simulink model "UAV_control"  (R2023a)
settings: Solver=FixedStepAuto  StartTime=0.0  StopTime=20  FixedStep=0.01  RelTol=1e-3
InitFcn:
  | parameters_UAV
values from neighbouring files (symbols this model uses):
  attitudeInit = [0;0;0]    [parameters_UAV.m]
  b = m*g/(4*w0r^2)    (= 1.31218568726e-05)    [parameters_UAV.m]
  d = 1.218100e-07    (= 1.2181e-07)    [parameters_UAV.m]
  g = 9.81    [parameters_UAV.m]
  I = diag([Ix, Iy, Iz])    [parameters_UAV.m]
  Jm = 12*10^-6    (= 1.2e-05)    [parameters_UAV.m]
  Ke = Kt    (= 0.00502594557132)    [parameters_UAV.m]
  Kp1P = Iy*etaP*wnP/(Kth*L)    (= 0.0922548996874)    [parameters_UAV.m]
  Kp1R = Ix*etaR*wnR/(Kth*L)    (= 0.0956695521884)    [parameters_UAV.m]
  Kp1x = 2*m*etax*wnx/U1    (= 0.203873598369)    [parameters_UAV.m]
  Kp1Y = Iz*etaY*wnY/(2*Kd)    (= 0.791166525164)    [parameters_UAV.m]
  Kp1y = 2*m*etay*wny/U1    (= 0.203873598369)    [parameters_UAV.m]
  Kp1z = m*etaz*wnz/(2*Kth)    (= 2.43380373272)    [parameters_UAV.m]
  Kp2P = Iy*wnP^2/(2*Kth*L*Kp1P)    (= 4.28571428571)    [parameters_UAV.m]
  Kp2R = Ix*wnR^2/(2*Kth*L*Kp1R)    (= 4.28571428571)    [parameters_UAV.m]
  Kp2x = m*wnx^2/(U1*Kp1x)    (= 0.5)    [parameters_UAV.m]
  Kp2Y = Iz*wnY^2/(4*Kd*Kp1Y)    (= 2.85714285714)    [parameters_UAV.m]
  Kp2y = m*wny^2/(U1*Kp1y)    (= 0.5)    [parameters_UAV.m]
  Kp2z = m*wnz^2/(4*Kth*Kp1z)    (= 0.333333333333)    [parameters_UAV.m]
  Kt = 1/(1900/60*2*pi)    (= 0.00502594557132)    [parameters_UAV.m]
  L = 0.211    [parameters_UAV.m]
  m = 1.362    [parameters_UAV.m]
  MotorSpeedInit = 0    [parameters_UAV.m]
  omegaInit = [0;0;0]    [parameters_UAV.m]
  posInit = [0;0;0]    [parameters_UAV.m]
  Ra = 0.128    [parameters_UAV.m]
  u0 = (w0-1075)/7525    (= 0.497408637874)    [parameters_UAV.m]
  velInit = [0;0;0]    [parameters_UAV.m]
settings Model: Creator=THETRUNG  LastModifiedBy=ducdu
settings SolverCC: AlgebraicLoopSolver=TrustRegion
settings OptimizationCC: UseRowMajorAlgorithm=on
settings DebuggingCC: UnconnectedInputMsg=warning  UnconnectedOutputMsg=warning  UnconnectedLineMsg=warning
settings ModelReferenceCC: EnableRefExpFcnMdlSchedulingChecks=on
settings SFSimCC: CustomCodeUndefinedFunction=UseInterfaceOnly

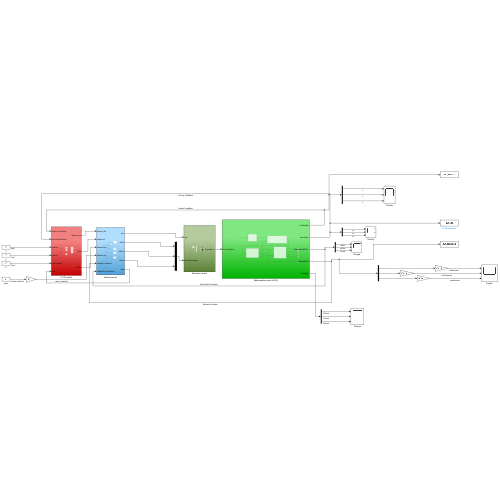
[thumbnail: Simulink's stored preview of the top-level diagram]
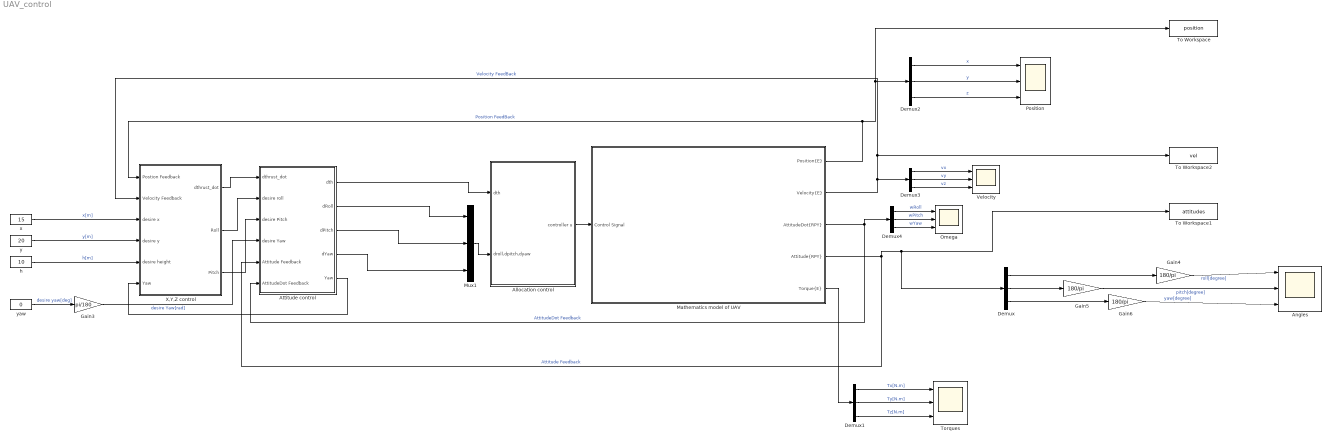
== system UAV_control ==
  "Allocation control " : Subsystem
  Angles : Scope  NumInputPorts=3
  Attitude control : Subsystem
  Demux{,1..4} (5 alike) : Demux  Outputs=3
  Gain3 : Gain  Gain=pi/180
  Gain4 : Gain  Gain=180/pi
  Gain5 : Gain  Gain=180/pi
  Gain6 : Gain  Gain=180/pi
  Mathematics model of UAV : Subsystem
  Mux1 : Mux  Inputs=3
  Omega : Scope  NumInputPorts=3
  Position : Scope  NumInputPorts=3
  To Workspace : ToWorkspace  VariableName=position  SampleTime=1
  To Workspace1 : ToWorkspace  VariableName=attitudes  SampleTime=1
  To Workspace2 : ToWorkspace  VariableName=vel  SampleTime=1
  Torques : Scope  NumInputPorts=3
  Velocity : Scope  NumInputPorts=3
  X,Y,Z control : Subsystem
  h : Constant  Value=10
  x : Constant  Value=15
  y : Constant  Value=20
  "yaw " : Constant  Value=0
  wires:
  Demux/1 -> Gain4/1
  Demux/2 -> Gain5/1
  Demux/3 -> Gain6/1
  Demux1/1 -> Torques/1  "Tx[N.m]"
  Demux1/2 -> Torques/2  "Ty[N.m]"
  Demux1/3 -> Torques/3  "Tz[N.m]"
  Demux2/3 -> Position/3  "z"
  Demux2/1 -> Position/1  "x"
  Demux2/2 -> Position/2  "y"
  "yaw "/1 -> Gain3/1  "desire yaw[deg]"
  Demux3/3 -> Velocity/3  "vz"
  Demux3/1 -> Velocity/1  "vx"
  Demux3/2 -> Velocity/2  "vy"
  Demux4/2 -> Omega/2  "wPitch"
  Demux4/1 -> Omega/1  "wRoll"
  Demux4/3 -> Omega/3  "wYaw"
  "Allocation control "/1("controller u ") -> Mathematics model of UAV/1(Control Signal)
  Mathematics model of UAV/1("Position{E} ") -> X,Y,Z control/1(Postion Feedback), Demux2/1, To Workspace/1  "Position FeedBack"
  Mathematics model of UAV/5("Torque{E} ") -> Demux1/1
  Mathematics model of UAV/2("Velocity{E} ") -> To Workspace2/1, X,Y,Z control/2(Velocity Feedback), Demux3/1  "Velocity FeedBack"
  Mathematics model of UAV/3("AttitudeDot{RPY} ") -> Demux4/1, Attitude control/6(AttitudeDot Feedback)  "AttitudeDot Feedback"
  Mux1/1 -> "Allocation control "/2("droll,dpitch,dyaw ")
  Mathematics model of UAV/4("Attitude{RPY}") -> To Workspace1/1, Demux/1, Attitude control/5(Attitude Feedback)  "Attitude Feedback"
  Attitude control/2(dRoll) -> Mux1/1
  Attitude control/3(dPitch) -> Mux1/2
  Attitude control/4(dYaw) -> Mux1/3
  X,Y,Z control/1(dthrust_dot) -> Attitude control/1(dthrust_dot)
  Gain4/1 -> Angles/1  "roll[degree]"
  Gain5/1 -> Angles/2  "pitch[degree]"
  Gain6/1 -> Angles/3  "yaw[degree]"
  x/1 -> X,Y,Z control/3(desire x)  "x[m]"
  y/1 -> X,Y,Z control/4(desire y)  "y[m]"
  h/1 -> X,Y,Z control/5(desire height)  "h[m]"
  Attitude control/1("dth ") -> "Allocation control "/1(dth)
  X,Y,Z control/2(Roll) -> Attitude control/2(desire roll)
  X,Y,Z control/3(Pitch) -> Attitude control/3(desire Pitch)
  Gain3/1 -> Attitude control/4(desire Yaw)  "desire Yaw[rad]"
  Attitude control/5(Yaw) -> X,Y,Z control/6(Yaw)

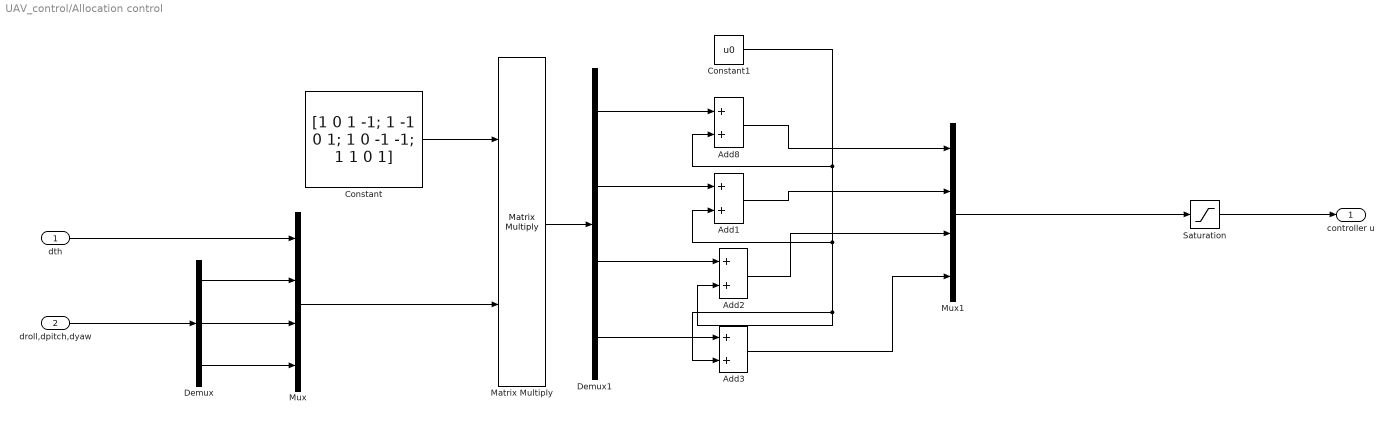
== system UAV_control/Allocation control  ==
  dth : Inport
  "droll,dpitch,dyaw " : Inport  Port=2
  Add{1..3,8} (4 alike) : Sum
  Constant : Constant  Value=[1 0 1 -1; 1 -1 0 1; 1 0 -1 -1; 1 1 0 1]
  Constant1 : Constant  Value=u0
  Demux : Demux  Outputs=3
  Demux1 : Demux
  Matrix Multiply : Product  Multiplication=Matrix(*)
  Mux : Mux
  Mux1 : Mux
  Saturation : Saturate  UpperLimit=1  LowerLimit=0
  "controller u " : Outport  VectorParamsAs1DForOutWhenUnconnected=off
  wires:
  "droll,dpitch,dyaw "/1 -> Demux/1
  Demux/3 -> Mux/4
  Demux/2 -> Mux/3
  Demux/1 -> Mux/2
  dth/1 -> Mux/1
  Constant/1 -> Matrix Multiply/1
  Mux/1 -> Matrix Multiply/2
  Matrix Multiply/1 -> Demux1/1
  Demux1/1 -> Add8/1
  Demux1/2 -> Add1/1
  Demux1/3 -> Add2/1
  Demux1/4 -> Add3/1
  Constant1/1 -> Add8/2, Add1/2, Add2/2, Add3/2
  Add8/1 -> Mux1/1
  Add1/1 -> Mux1/2
  Add2/1 -> Mux1/3
  Add3/1 -> Mux1/4
  Mux1/1 -> Saturation/1
  Saturation/1 -> "controller u "/1

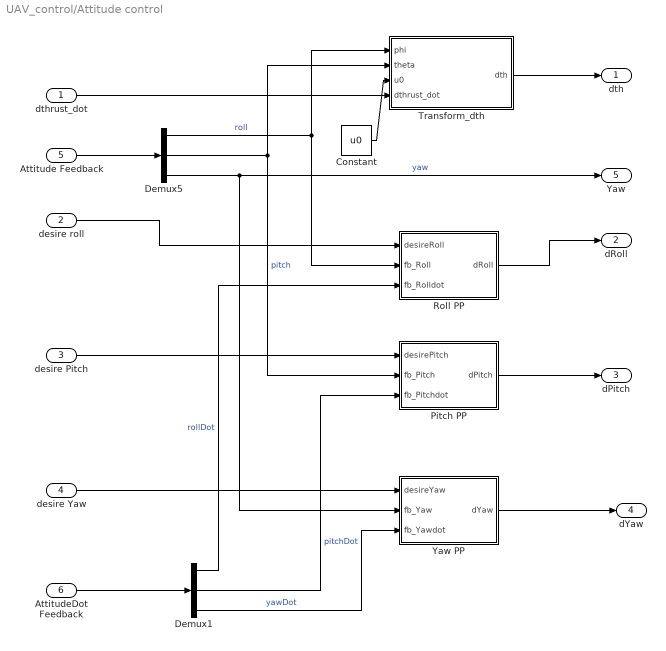
== system UAV_control/Attitude control ==
  dthrust_dot : Inport
  desire roll : Inport  Port=2
  desire Pitch : Inport  Port=3
  desire Yaw : Inport  Port=4
  Attitude Feedback : Inport  Port=5
  AttitudeDot Feedback : Inport  Port=6
  Constant : Constant  Value=u0
  Demux1 : Demux  Outputs=3
  Demux5 : Demux  Outputs=3
  Pitch PP : Subsystem
  "Roll PP " : Subsystem
  Transform_dth : MATLAB Function  TreatAsAtomicUnit=on
  Yaw PP : Subsystem
  "dth " : Outport  VectorParamsAs1DForOutWhenUnconnected=off
  dRoll : Outport  Port=2  VectorParamsAs1DForOutWhenUnconnected=off
  dPitch : Outport  Port=3  VectorParamsAs1DForOutWhenUnconnected=off
  dYaw : Outport  Port=4  VectorParamsAs1DForOutWhenUnconnected=off
  Yaw : Outport  Port=5  VectorParamsAs1DForOutWhenUnconnected=off
  wires:
  Demux5/3 -> Yaw/1, Yaw PP/2(fb_Yaw)  "yaw"
  Demux5/1 -> Transform_dth/1(phi), "Roll PP "/2(fb_Roll)  "roll"
  desire roll/1 -> "Roll PP "/1("desireRoll ")
  Demux5/2 -> Transform_dth/2(theta), Pitch PP/2(fb_Pitch)  "pitch"
  Attitude Feedback/1 -> Demux5/1
  "Roll PP "/1("dRoll ") -> dRoll/1
  Pitch PP/1("dPitch ") -> dPitch/1
  Yaw PP/1("dYaw ") -> dYaw/1
  desire Pitch/1 -> Pitch PP/1("desirePitch ")
  desire Yaw/1 -> Yaw PP/1("desireYaw ")
  Demux1/1 -> "Roll PP "/3(fb_Rolldot)  "rollDot"
  AttitudeDot Feedback/1 -> Demux1/1
  Demux1/3 -> Yaw PP/3(fb_Yawdot)  "yawDot"
  Demux1/2 -> Pitch PP/3(fb_Pitchdot)  "pitchDot"
  Transform_dth/1(dth) -> "dth "/1
  dthrust_dot/1 -> Transform_dth/4(dthrust_dot)
  Constant/1 -> Transform_dth/3(u0)

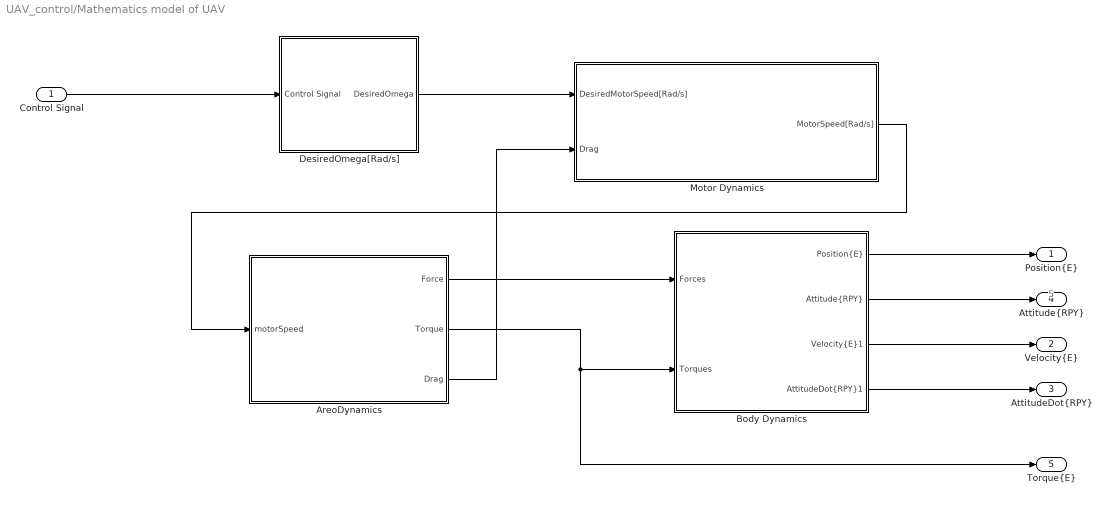
== system UAV_control/Mathematics model of UAV ==
  note: 5
  Control Signal : Inport
  "AreoDynamics " : Subsystem
  "Body Dynamics " : Subsystem
  DesiredOmega[Rad/s] : Subsystem
  Motor Dynamics : Subsystem
  "Position{E} " : Outport  VectorParamsAs1DForOutWhenUnconnected=off
  "Velocity{E} " : Outport  Port=2  VectorParamsAs1DForOutWhenUnconnected=off
  "AttitudeDot{RPY} " : Outport  Port=3  VectorParamsAs1DForOutWhenUnconnected=off
  "Attitude{RPY}" : Outport  Port=4  VectorParamsAs1DForOutWhenUnconnected=off
  "Torque{E} " : Outport  Port=5  VectorParamsAs1DForOutWhenUnconnected=off
  wires:
  "AreoDynamics "/1(Force) -> "Body Dynamics "/1("Forces ")
  Control Signal/1 -> DesiredOmega[Rad/s]/1(Control Signal)
  Motor Dynamics/1(MotorSpeed[Rad/s]) -> "AreoDynamics "/1(motorSpeed)
  "AreoDynamics "/2(Torque) -> "Torque{E} "/1, "Body Dynamics "/2("Torques ")
  "Body Dynamics "/4("AttitudeDot{RPY}1") -> "AttitudeDot{RPY} "/1
  DesiredOmega[Rad/s]/1(DesiredOmega) -> Motor Dynamics/1(DesiredMotorSpeed[Rad/s])
  "Body Dynamics "/2("Attitude{RPY}") -> "Attitude{RPY}"/1
  "AreoDynamics "/3("Drag ") -> Motor Dynamics/2("Drag ")
  "Body Dynamics "/1("Position{E}") -> "Position{E} "/1
  "Body Dynamics "/3("Velocity{E}1") -> "Velocity{E} "/1

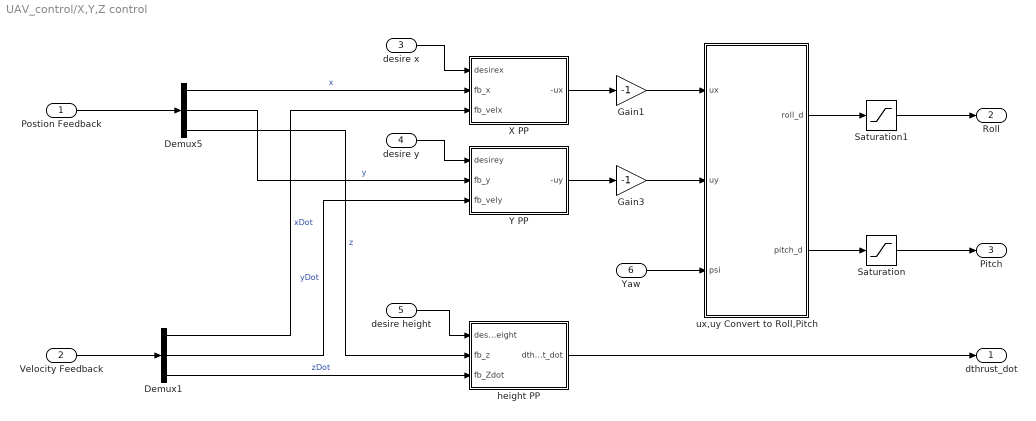
== system UAV_control/X,Y,Z control ==
  Postion Feedback : Inport
  Velocity Feedback : Inport  Port=2
  desire x : Inport  Port=3
  desire y : Inport  Port=4
  desire height : Inport  Port=5
  Yaw : Inport  Port=6
  Demux1 : Demux  Outputs=3
  Demux5 : Demux  Outputs=3
  Gain1 : Gain  Gain=-1  ParamDataTypeStr=double
  Gain3 : Gain  Gain=-1  ParamDataTypeStr=double
  Saturation : Saturate  UpperLimit=pi/8  LowerLimit=-pi/8
  Saturation1 : Saturate  UpperLimit=pi/8  LowerLimit=-pi/8
  "X PP " : Subsystem
  "Y PP " : Subsystem
  "height PP " : Subsystem
  ux,uy Convert to Roll,Pitch : MATLAB Function  TreatAsAtomicUnit=on
  dthrust_dot : Outport  VectorParamsAs1DForOutWhenUnconnected=off
  Roll : Outport  Port=2  OutDataTypeStr=double  VectorParamsAs1DForOutWhenUnconnected=off
  Pitch : Outport  Port=3  OutDataTypeStr=double  VectorParamsAs1DForOutWhenUnconnected=off
  wires:
  Demux5/3 -> "height PP "/2(fb_z)  "z"
  Demux5/1 -> "X PP "/2(fb_x)  "x"
  desire x/1 -> "X PP "/1("desirex ")
  Demux5/2 -> "Y PP "/2(fb_y)  "y"
  Postion Feedback/1 -> Demux5/1
  "Y PP "/1("-uy ") -> Gain3/1
  "height PP "/1("dthrust_dot ") -> dthrust_dot/1
  desire y/1 -> "Y PP "/1("desirey ")
  desire height/1 -> "height PP "/1("desireHeight ")
  Demux1/1 -> "X PP "/3(fb_velx)  "xDot"
  Velocity Feedback/1 -> Demux1/1
  Demux1/3 -> "height PP "/3(fb_Zdot)  "zDot"
  Demux1/2 -> "Y PP "/3(fb_vely)  "yDot"
  Gain3/1 -> ux,uy Convert to Roll,Pitch/2(uy)
  Yaw/1 -> ux,uy Convert to Roll,Pitch/3(psi)
  Saturation1/1 -> Roll/1
  Saturation/1 -> Pitch/1
  "X PP "/1("-ux ") -> Gain1/1
  ux,uy Convert to Roll,Pitch/1(roll_d) -> Saturation1/1
  ux,uy Convert to Roll,Pitch/2(pitch_d) -> Saturation/1
  Gain1/1 -> ux,uy Convert to Roll,Pitch/1(ux)

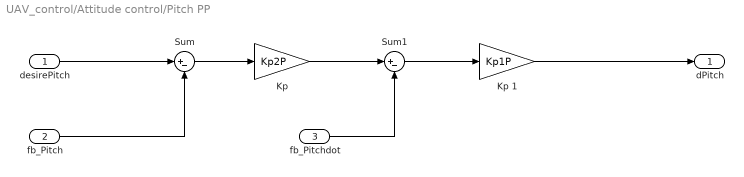
== system UAV_control/Attitude control/Pitch PP ==
  "desirePitch " : Inport
  fb_Pitch : Inport  Port=2
  fb_Pitchdot : Inport  Port=3
  "Kp " : Gain  Gain=Kp2P
  Kp 1 : Gain  Gain=Kp1P
  Sum : Sum  Inputs=|+-
  Sum1 : Sum  Inputs=|+-
  "dPitch " : Outport  VectorParamsAs1DForOutWhenUnconnected=off
  wires:
  "desirePitch "/1 -> Sum/1
  fb_Pitch/1 -> Sum/2
  Sum/1 -> "Kp "/1
  "Kp "/1 -> Sum1/1
  Sum1/1 -> Kp 1/1
  Kp 1/1 -> "dPitch "/1
  fb_Pitchdot/1 -> Sum1/2

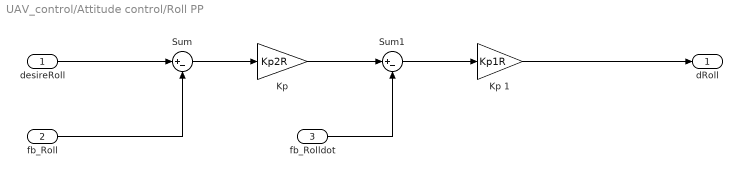
== system UAV_control/Attitude control/Roll PP  ==
  "desireRoll " : Inport
  fb_Roll : Inport  Port=2
  fb_Rolldot : Inport  Port=3
  "Kp " : Gain  Gain=Kp2R
  Kp 1 : Gain  Gain=Kp1R
  Sum : Sum  Inputs=|+-
  Sum1 : Sum  Inputs=|+-
  "dRoll " : Outport  VectorParamsAs1DForOutWhenUnconnected=off
  wires:
  "desireRoll "/1 -> Sum/1
  fb_Roll/1 -> Sum/2
  Sum/1 -> "Kp "/1
  "Kp "/1 -> Sum1/1
  Sum1/1 -> Kp 1/1
  Kp 1/1 -> "dRoll "/1
  fb_Rolldot/1 -> Sum1/2

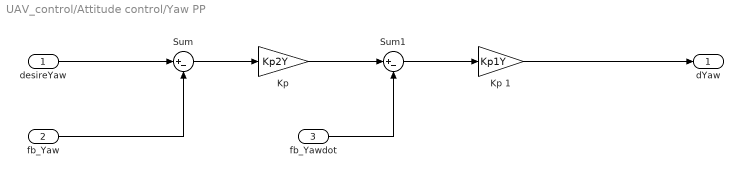
== system UAV_control/Attitude control/Yaw PP ==
  "desireYaw " : Inport
  fb_Yaw : Inport  Port=2
  fb_Yawdot : Inport  Port=3
  "Kp " : Gain  Gain=Kp2Y
  Kp 1 : Gain  Gain=Kp1Y
  Sum : Sum  Inputs=|+-
  Sum1 : Sum  Inputs=|+-
  "dYaw " : Outport  VectorParamsAs1DForOutWhenUnconnected=off
  wires:
  "desireYaw "/1 -> Sum/1
  fb_Yaw/1 -> Sum/2
  Sum/1 -> "Kp "/1
  "Kp "/1 -> Sum1/1
  Sum1/1 -> Kp 1/1
  Kp 1/1 -> "dYaw "/1
  fb_Yawdot/1 -> Sum1/2

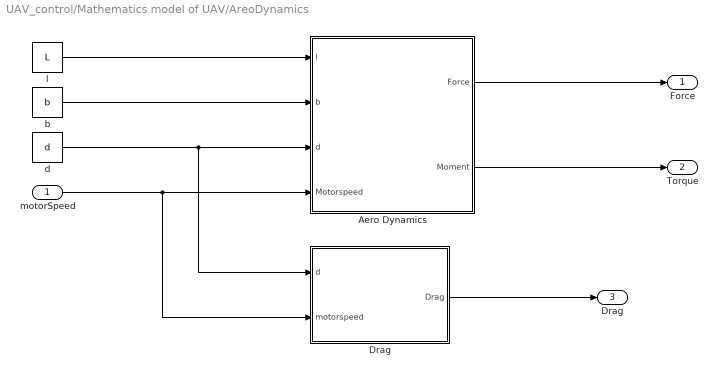
== system UAV_control/Mathematics model of UAV/AreoDynamics  ==
  motorSpeed : Inport
  "Aero Dynamics " : MATLAB Function  TreatAsAtomicUnit=on
  "Drag " : MATLAB Function  TreatAsAtomicUnit=on
  b : Constant  Value=b
  d : Constant  Value=d
  l : Constant  Value=L
  Force : Outport  VectorParamsAs1DForOutWhenUnconnected=off
  Torque : Outport  Port=2  VectorParamsAs1DForOutWhenUnconnected=off
  "Drag " : Outport  Port=3  VectorParamsAs1DForOutWhenUnconnected=off
  wires:
  "Aero Dynamics "/1(Force) -> Force/1
  "Aero Dynamics "/2(Moment) -> Torque/1
  motorSpeed/1 -> "Drag "/2(motorspeed), "Aero Dynamics "/4(Motorspeed)
  b/1 -> "Aero Dynamics "/2(b)
  l/1 -> "Aero Dynamics "/1(l)
  d/1 -> "Drag "/1(d), "Aero Dynamics "/3(d)
  "Drag "/1(Drag) -> "Drag "/1

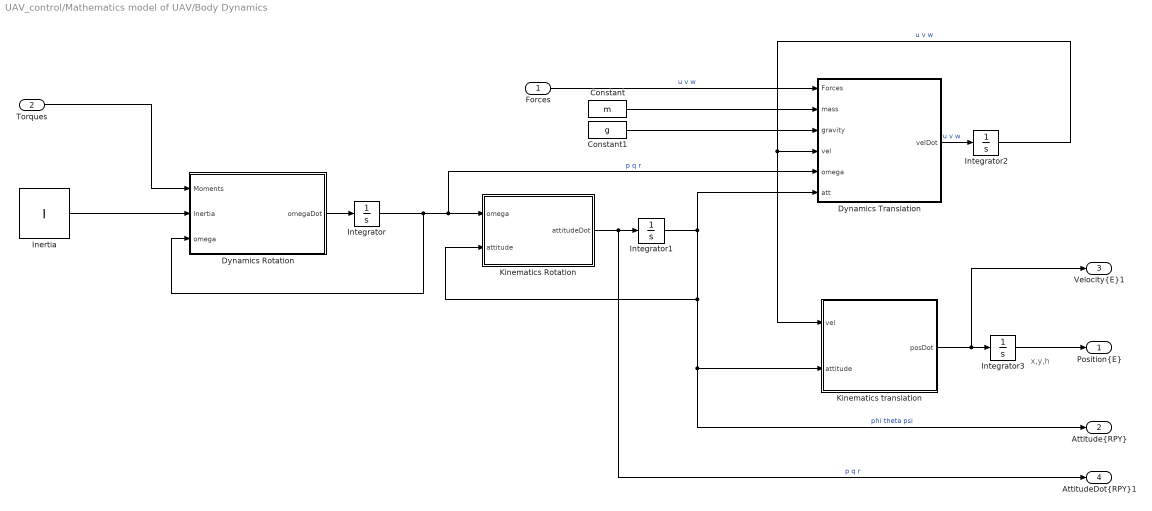
== system UAV_control/Mathematics model of UAV/Body Dynamics  ==
  note: x,y,h
  "Forces " : Inport
  "Torques " : Inport  Port=2
  Constant : Constant  Value=m
  Constant1 : Constant  Value=g
  "Dynamics Rotation " : MATLAB Function  TreatAsAtomicUnit=on
  "Dynamics Translation " : MATLAB Function  TreatAsAtomicUnit=on
  "Inertia " : Constant  Value=I
  Integrator : Integrator  InitialCondition=omegaInit
  Integrator1 : Integrator  InitialCondition=attitudeInit
  Integrator2 : Integrator  InitialCondition=velInit
  Integrator3 : Integrator  InitialCondition=posInit
  "Kinematics Rotation " : MATLAB Function  TreatAsAtomicUnit=on
  "Kinematics translation " : MATLAB Function  TreatAsAtomicUnit=on
  "Position{E}" : Outport  VectorParamsAs1DForOutWhenUnconnected=off
  "Attitude{RPY}" : Outport  Port=2  VectorParamsAs1DForOutWhenUnconnected=off
  "Velocity{E}1" : Outport  Port=3  VectorParamsAs1DForOutWhenUnconnected=off
  "AttitudeDot{RPY}1" : Outport  Port=4  VectorParamsAs1DForOutWhenUnconnected=off
  wires:
  Integrator3/1 -> "Position{E}"/1
  Constant/1 -> "Dynamics Translation "/2(mass)
  Integrator/1 -> "Dynamics Translation "/5(omega), "Kinematics Rotation "/1(omega), "Dynamics Rotation "/3(omega)  "p q r"
  Constant1/1 -> "Dynamics Translation "/3(gravity)
  "Torques "/1 -> "Dynamics Rotation "/1(Moments)
  Integrator1/1 -> "Dynamics Translation "/6(att), "Attitude{RPY}"/1, "Kinematics translation "/2(attitude), "Kinematics Rotation "/2(attitude)  "phi theta psi"
  Integrator2/1 -> "Kinematics translation "/1(vel), "Dynamics Translation "/4(vel)  "u v w"
  "Inertia "/1 -> "Dynamics Rotation "/2(Inertia)
  "Kinematics translation "/1(posDot) -> Integrator3/1, "Velocity{E}1"/1
  "Dynamics Rotation "/1(omegaDot) -> Integrator/1
  "Forces "/1 -> "Dynamics Translation "/1(Forces)  "u v w"
  "Dynamics Translation "/1(velDot) -> Integrator2/1  "u v w"
  "Kinematics Rotation "/1(attitudeDot) -> Integrator1/1, "AttitudeDot{RPY}1"/1  "p q r"

== system UAV_control/Mathematics model of UAV/DesiredOmega[Rad//s] ==
  Control Signal : Inport
  PWM2RPM : MATLAB Function  TreatAsAtomicUnit=on
  RPM2Radps : MATLAB Function  TreatAsAtomicUnit=on
  DesiredOmega : Outport  VectorParamsAs1DForOutWhenUnconnected=off
  wires:
  Control Signal/1 -> PWM2RPM/1(u)
  PWM2RPM/1(RPM) -> RPM2Radps/1(RPM)
  RPM2Radps/1(Radps) -> DesiredOmega/1

== system UAV_control/Mathematics model of UAV/Motor Dynamics ==
  DesiredMotorSpeed[Rad/s] : Inport
  "Drag " : Inport  Port=2
  MotorDynamics : Subsystem
  SpeedVoltageConversion : Subsystem
  MotorSpeed[Rad/s] : Outport  VectorParamsAs1DForOutWhenUnconnected=off
  wires:
  MotorDynamics/1(MotorSpeed[Rad/s]) -> MotorSpeed[Rad/s]/1
  DesiredMotorSpeed[Rad/s]/1 -> SpeedVoltageConversion/1(DesignMotorSpeed)
  "Drag "/1 -> MotorDynamics/2(DragTorque)
  SpeedVoltageConversion/1("MotorVoltage ") -> MotorDynamics/1(Voltage[V])

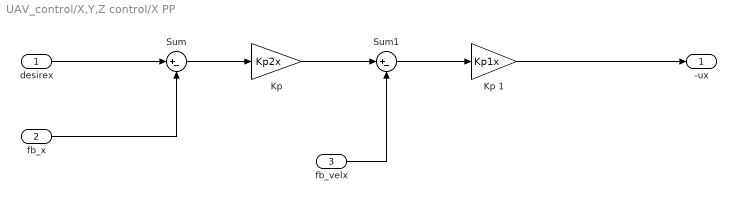
== system UAV_control/X,Y,Z control/X PP  ==
  "desirex " : Inport
  fb_x : Inport  Port=2
  fb_velx : Inport  Port=3
  "Kp " : Gain  Gain=Kp2x
  Kp 1 : Gain  Gain=Kp1x
  Sum : Sum  Inputs=|+-
  Sum1 : Sum  Inputs=|+-
  "-ux " : Outport  VectorParamsAs1DForOutWhenUnconnected=off
  wires:
  "desirex "/1 -> Sum/1
  fb_x/1 -> Sum/2
  Sum/1 -> "Kp "/1
  "Kp "/1 -> Sum1/1
  Sum1/1 -> Kp 1/1
  Kp 1/1 -> "-ux "/1
  fb_velx/1 -> Sum1/2

== system UAV_control/X,Y,Z control/Y PP  ==
  "desirey " : Inport
  fb_y : Inport  Port=2
  fb_vely : Inport  Port=3
  "Kp " : Gain  Gain=Kp2y
  Kp 1 : Gain  Gain=Kp1y
  Sum : Sum  Inputs=|+-
  Sum1 : Sum  Inputs=|+-
  "-uy " : Outport  VectorParamsAs1DForOutWhenUnconnected=off
  wires:
  "desirey "/1 -> Sum/1
  fb_y/1 -> Sum/2
  Sum/1 -> "Kp "/1
  "Kp "/1 -> Sum1/1
  Sum1/1 -> Kp 1/1
  Kp 1/1 -> "-uy "/1
  fb_vely/1 -> Sum1/2

== system UAV_control/X,Y,Z control/height PP  ==
  "desireHeight " : Inport
  fb_z : Inport  Port=2
  fb_Zdot : Inport  Port=3
  "Kp " : Gain  Gain=Kp2z
  Kp 1 : Gain  Gain=Kp1z
  Sum : Sum  Inputs=|++
  Sum1 : Sum  Inputs=|++
  "dthrust_dot " : Outport  VectorParamsAs1DForOutWhenUnconnected=off
  wires:
  fb_z/1 -> Sum/2
  Sum/1 -> "Kp "/1
  "Kp "/1 -> Sum1/1
  Sum1/1 -> Kp 1/1
  Kp 1/1 -> "dthrust_dot "/1
  "desireHeight "/1 -> Sum/1
  fb_Zdot/1 -> Sum1/2

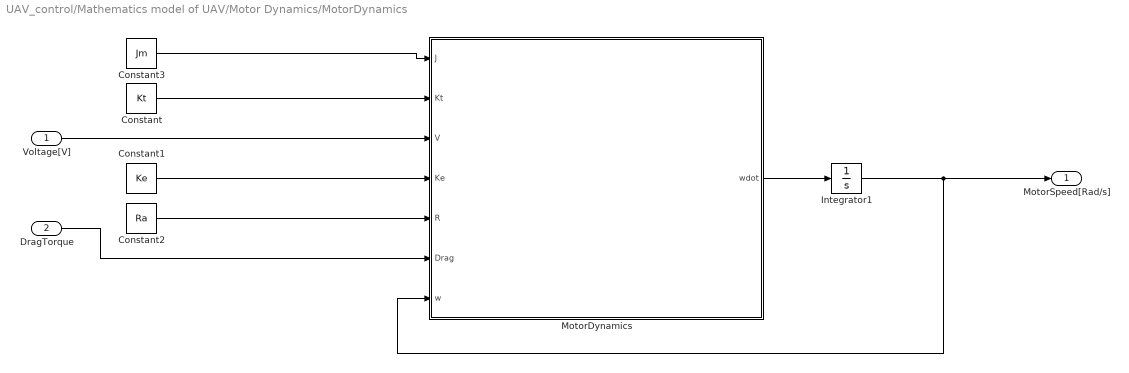
== system UAV_control/Mathematics model of UAV/Motor Dynamics/MotorDynamics ==
  Voltage[V] : Inport
  DragTorque : Inport  Port=2
  Constant : Constant  Value=Kt
  Constant1 : Constant  Value=Ke
  Constant2 : Constant  Value=Ra
  Constant3 : Constant  Value=Jm
  Integrator1 : Integrator  InitialCondition=MotorSpeedInit
  MotorDynamics : MATLAB Function  TreatAsAtomicUnit=on
  MotorSpeed[Rad/s] : Outport  VectorParamsAs1DForOutWhenUnconnected=off
  wires:
  Voltage[V]/1 -> MotorDynamics/3(V)
  Constant/1 -> MotorDynamics/2(Kt)
  Constant1/1 -> MotorDynamics/4(Ke)
  Constant2/1 -> MotorDynamics/5(R)
  DragTorque/1 -> MotorDynamics/6(Drag)
  MotorDynamics/1(wdot) -> Integrator1/1
  Constant3/1 -> MotorDynamics/1(J)
  Integrator1/1 -> MotorSpeed[Rad/s]/1, MotorDynamics/7(w)

== system UAV_control/Mathematics model of UAV/Motor Dynamics/SpeedVoltageConversion ==
  DesignMotorSpeed : Inport
  Constant : Constant  Value=Ra
  Constant1 : Constant  Value=Ke
  Constant2 : Constant  Value=Kt
  Constant3 : Constant  Value=d
  Converter : MATLAB Function  TreatAsAtomicUnit=on
  Saturation : Saturate  UpperLimit=12  LowerLimit=0
  "MotorVoltage " : Outport  VectorParamsAs1DForOutWhenUnconnected=off
  wires:
  DesignMotorSpeed/1 -> Converter/5(wdesign)
  Converter/1(V) -> Saturation/1
  Constant3/1 -> Converter/4(d)
  Constant2/1 -> Converter/3(Kt)
  Constant/1 -> Converter/2(Ra)
  Constant1/1 -> Converter/1(Ke)
  Saturation/1 -> "MotorVoltage "/1

== matlab function UAV_control/Mathematics model of UAV/AreoDynamics /Drag  ==
  data: d input; motorspeed input; Drag output
function Drag = fcn(d,motorspeed)
Drag = eye(4,1)*0;
Drag =d*motorspeed.^2.*sign(motorspeed);
end

== matlab function UAV_control/X,Y,Z control/ux,uy Convert to Roll,Pitch ==
  data: ux input; roll_d output; uy input; psi input; pitch_d output
% function [phi, theta]= fcn(ux,uy, psi)
%     A = ux*sin(psi) - uy*cos(psi);
%     A(A>1) = 1;
%     A(A<-1) = -1;
%     phi = asin(A);
%     B = (ux*cos(psi)-uy*sin(psi))/cos(phi);
%     B(B>1) = 1;
%     B(B<-1) = -1;
%     theta = asin(B);
% end
function [roll_d, pitch_d] = fcn(ux,uy,psi)
sin_roll_d = ux*sin(psi) - uy*cos(psi);
sin_roll_d = max(min(sin_roll_d,1),-1);
roll_d = asin(sin_roll_d);
sin_pitch_d = (ux*cos(psi)+uy*sin(psi))/cos(roll_d);
sin_pitch_d = max(min(sin_pitch_d,1),-1);
pitch_d = asin(sin_pitch_d);

== matlab function UAV_control/Attitude control/Transform_dth ==
  data: phi input; dth output; theta input; u0 input; dthrust_dot input
function dth = fcn(phi, theta, u0,dthrust_dot)

dth = (u0+dthrust_dot)/(cos(phi)*cos(theta)) - u0;

== matlab function UAV_control/Mathematics model of UAV/Body Dynamics /Kinematics Rotation  ==
  data: omega input; attitudeDot output; attitude input
function attitudeDot = fcn(omega,attitude)
phi = attitude(1);
theta = attitude(2);

WB_E = [1 sin(phi)*tan(theta) cos(phi)*tan(theta);
        0        cos(phi)            -sin(phi);
        0   sin(phi)/cos(theta) cos(phi)/cos(theta)];
attitudeDot = WB_E*omega;    
end

== matlab function UAV_control/Mathematics model of UAV/Body Dynamics /Kinematics translation  ==
  data: vel input; posDot output; attitude input
function posDot = fcn(vel,attitude)
phi = attitude(1);
theta = attitude(2);
psi = attitude(3);

RB_E = [cos(theta)*cos(psi) sin(phi)*sin(theta)*cos(psi)-cos(phi)*sin(psi) cos(phi)*sin(theta)*cos(psi)+sin(phi)*sin(psi);
     cos(theta)*sin(psi) sin(phi)*sin(theta)*sin(psi)+cos(phi)*cos(psi) cos(phi)*sin(theta)*sin(psi)-sin(phi)*cos(psi);
          -sin(theta)                                sin(phi)*cos(theta)                      cos(phi)*cos(theta)];
posDot = RB_E*vel;
end

== matlab function UAV_control/Mathematics model of UAV/Body Dynamics /Dynamics Translation  ==
  data: Forces input; mass input; gravity input; vel input; velDot output; omega input; att input
function velDot = fcn(Forces,mass,gravity,vel,omega,att)
wb = omega;
attitude = att;

phi = attitude(1);
theta = attitude(2);

g = [-gravity*sin(theta);
    gravity*sin(phi)*cos(theta);
    gravity*cos(phi)*cos(theta)];
        
velDot = 1/mass*Forces + g - cross(wb,vel);
end

== matlab function UAV_control/Mathematics model of UAV/Body Dynamics /Dynamics Rotation  ==
  data: Moments input; Inertia input; omegaDot output; omega input
function omegaDot = fcn(Moments,Inertia,omega)
J = Inertia;
wb = omega;
T = Moments;
omegaDot = J^(-1)*(T - cross(wb,J*wb));
end

== matlab function UAV_control/Mathematics model of UAV/Motor Dynamics/MotorDynamics/MotorDynamics ==
  data: J input; Kt input; wdot output; V input; Ke input; R input; Drag input; w input
function wdot = fcn(J,Kt,V,Ke,R,Drag,w)
    I = (V-Ke*w)/R;
    wdot = (Kt*I -Drag)/J;
    threshold = 10^-2;
    wdot(abs(wdot)<threshold) = 0;
end

== matlab function UAV_control/Mathematics model of UAV/AreoDynamics /Aero Dynamics  ==
  data: l input; b input; d input; Force output; Motorspeed input; Moment output
function [Force,Moment] = fcn(l, b, d, Motorspeed)
omega1 = Motorspeed(1);
omega2 = Motorspeed(2);
omega3 = Motorspeed(3);
omega4 = Motorspeed(4);
Force = [0;
    0;
    -b*(omega1^2 + omega2^2 + omega3^2 + omega4^2)];

Moment = [  l*b*(omega4^2 - omega2^2);
            l*b*(omega1^2 - omega3^2);
            d*(-omega1^2 + omega2^2 - omega3^2 + omega4^2)];
threshold = 10^-8;
Force(abs(Force)<threshold) = 0;
Moment(abs(Moment)<threshold) = 0;
end

== matlab function UAV_control/Mathematics model of UAV/Motor Dynamics/SpeedVoltageConversion/Converter ==
  data: Ke input; V output; Ra input; Kt input; d input; wdesign input
function V = fcn(Ke,Ra,Kt,d,wdesign)
    V = Ke*wdesign + (d*Ra/Kt)*wdesign.^2;
end

== matlab function UAV_control/Mathematics model of UAV/DesiredOmega[Rad//s]/PWM2RPM ==
  data: u input; RPM output
function RPM = fcn(u)
    RPM = 1075 + 7525*u;
end

== matlab function UAV_control/Mathematics model of UAV/DesiredOmega[Rad//s]/RPM2Radps ==
  data: RPM input; Radps output
function Radps = fcn(RPM)
    Radps = RPM*(2*pi)/60;
end
